simulink library "ddm"  (R2021b)
settings: Solver=VariableStepAuto  StartTime=0.0  StopTime=10.0  RelTol=1e-3
undefined symbols (not defined in the file or in its folder): ADDM_FrTMTqDev_X_Nm, ADDM_RrTMTqDev_X_Nm, ENUM_ADASACCSTA_ERROR, ENUM_ADASACCSTA_OFF, ENUM_ADASACCSTA_STANDBY, ENUM_ALLOWMOV_ALLOWREADY, ENUM_APS, ENUM_BRKSTA_ERROR, ENUM_BRKSTA_OFF, ENUM_BRKSTA_ON, ENUM_BRKSW_INVALID, ENUM_BRKSW_OFF, ENUM_BRKSW_ON, ENUM_CHGPREACTERRSTA_OBCPRE, ENUM_DCDCFAULTSTA_ANYFAULTLV1, ENUM_DCDCFAULTSTA_ANYFAULTLV2, ENUM_DRIVETRAIN_AWD, ENUM_DRIVETRAIN_FWD, ENUM_DRIVETRAIN_RWD, ENUM_EDUDRTSTA_NORMAL, ENUM_EPBSTA_APPLIED, ENUM_EPBSTA_RELEASED, ENUM_ESCAPSSta_APSUNAVAILABLE, ENUM_GEARACTUALPOSN_INVALID, ENUM_GEARACTUALPOSN_P, ENUM_HVBATTREADYPRE_READY, ENUM_MCUWARN_LV0, ENUM_MCUWARN_LV1, ENUM_MCUWARN_LV2, ENUM_MCUWARN_LV3, ENUM_MCUWARN_NOERROR, ENUM_OBCFAULTSTA_ANYFAULT, ENUM_PAS_R2F2, ENUM_PDFAULT_BATTPDFAIL, ENUM_PDFAULT_DCDCDISABLE, ENUM_PDFAULT_MCUDISABLE, ENUM_PDFAULT_MCUDISCHRG, ENUM_POWERSTA_OFF, ENUM_POWERSTA_ON, ENUM_POWERSTA_READY, ENUM_POWERSTA_STANDBY, ENUM_PRESSINDI_LOW, ENUM_PUFAULT_BATTUPFAIL, ENUM_PUFAULT_DCDCENABLEFAIL, ENUM_PUFAULT_PRECHRGCHKFAIL, ENUM_PUFAULT_SAFETYCHKFAIL, ENUM_PUSTATE_COMPLETED, ENUM_PWRSTASW_OFF, ENUM_PWRSTASW_OFFA, ENUM_PWRSTASW_OFFCHVCHRG, ENUM_PWRSTASW_OFFCLVCHRG, ENUM_PWRSTASW_ON, ENUM_PWRSTASW_ONHVCHRG, ENUM_PWRSTASW_READY, ENUM_PWRSTASW_STANDBY, ENUM_RAPSErrWarnSta_NORMAL, ENUM_RAPSErrWarnSta_RAPSERRLV1, ENUM_SHIFTCOMMAND_P, ENUM_SHIFTERERRSTA_PBUTTONFAILURE, ENUM_VEHMALFUNLV_2ND ... (+463)
libraries: hcu_lib x529, $bdroot x5, simulink x4
(part 13 of 25)

== system ddm/DDM/DDM/TQD/ESC1_DDM ==
  note: Diagnostics and Fault Handling
  note: Release Condition After Decision
  note: Release Condition After Decision
  note: Diagnostics and Fault Handling
  note: Diagnostics and Fault Handling
  note: Release Condition After Decision
  note: ESC1 CheckSum Error (ESC1CSErr)
  note: ESC1 Rolling Count Error (ESC1RCErr)
  note: ESC1 Lost Comm (ESC1NoCom)
  task_time_s : Inport
  VPMM_SysPwrSta_enum : Inport  Port=2
  No_CAN1_BUS_OFF : Inport  Port=3
  VDDM_ESC1NoCom_flg : Inport  Port=4
  VDDM_ESC1RCErr_flg : Inport  Port=5
  VDDM_ESC1CSErr_flg : Inport  Port=6
  DTC_clear_request : Inport  Port=7
  Constant{1,3..5,11,15,19..20,48} (9 alike) : Constant  Value=ENUM_PWRSTASW_OFF
  Constant10 : Constant  Value=KDDM_TQDDiagnosisOffSW_flg
  Constant101 : Constant  Value=KDDM_TQDDiagnosisOffSW_flg
  Constant102 : Constant  Value=ZERO_INT
  Constant12 : Constant  Value=FALSE
  Constant13 : Constant  Value=KDDM_ESC1RCErrDTC_cnt
  Constant14 : Constant  Value=KDDM_ESC1RCErrPassTO_s
  Constant16 : Constant  Value=KDDM_ESC1CSErrDTC_cnt
  Constant17 : Constant  Value=KDDM_TQDDiagnosisOffSW_flg
  Constant18 : Constant  Value=ENUM_PWRSTASW_STANDBY
  Constant2 : Constant  Value=KDDM_ESC1NoComDTC_cnt
  Constant25 : Constant  Value=KDDM_ESC1RCErrDetTO_s
  Constant27 : Constant  Value=FALSE
  Constant28 : Constant  Value=KDDM_ESC1NoComDTC_cnt
  Constant29 : Constant  Value=KDDM_ESC1NoComPassTO_s
  Constant30 : Constant  Value=KDDM_ESC1NoComDetTO_s
  Constant35 : Constant  Value=KDDM_ESC1RCErrPassTO_s
  Constant41 : Constant  Value=FALSE
  Constant42 : Constant  Value=KDDM_ESC1CSErrDTC_cnt
  Constant43 : Constant  Value=KDDM_ESC1CSErrPassTO_s
  Constant44 : Constant  Value=KDDM_ESC1CSErrDetTO_s
  Constant45 : Constant  Value=ZERO_INT
  Constant51 : Constant  Value=KDDM_ESC1CSErrPassTO_s
  Constant55 : Constant  Value=KDDM_ESC1NoComPassTO_s
  Constant6 : Constant  Value=KDDM_ESC1RCErrDTC_cnt
  Constant7 : Constant  Value=ZERO_INT
  Constant8 : Constant  Value=ENUM_PWRSTASW_STANDBY
  Constant9 : Constant  Value=ENUM_PWRSTASW_STANDBY
  DTC_Couter1 : hcu_lib/Basic_Blocks/DTC_Couter
  DTC_Couter2 : hcu_lib/Basic_Blocks/DTC_Couter
  DTC_Couter7 : hcu_lib/Basic_Blocks/DTC_Couter
  DTC_Info1 : hcu_lib/Basic_Blocks/DTC_Info
  DTC_Info2 : hcu_lib/Basic_Blocks/DTC_Info
  DTC_Info3 : hcu_lib/Basic_Blocks/DTC_Info
  Delay1 : Delay  DelayLength=1
  Delay2 : Delay  DelayLength=1
  Delay3 : Delay  DelayLength=1
  Equal{1,7,9..10,49..50} (6 alike) : RelationalOperator  Operator===  OutDataTypeStr=boolean  RndMeth=Simplest
  Equal{2..4,6,8,11} (6 alike) : RelationalOperator  Operator=~=  OutDataTypeStr=boolean  RndMeth=Simplest
  Equal15 : RelationalOperator  OutDataTypeStr=boolean  RndMeth=Simplest
  Equal20 : RelationalOperator  OutDataTypeStr=boolean  RndMeth=Simplest
  Equal21 : RelationalOperator  OutDataTypeStr=boolean  RndMeth=Simplest
  Logical Operator : Logic  Operator=OR  Inputs=3  AllPortsSameDT=off  OutDataTypeStr=boolean
  Logical Operator1 : Logic  Operator=OR  Inputs=4  AllPortsSameDT=off  OutDataTypeStr=boolean
  Logical Operator{11..13,19,26,30,37,41,45,53} (10 alike) : Logic  Operator=NOT  AllPortsSameDT=off  OutDataTypeStr=boolean
  Logical Operator{2,5,8..9,14,49} (6 alike) : Logic  AllPortsSameDT=off  OutDataTypeStr=boolean
  Logical Operator{28,32,43,46} (4 alike) : Logic  Inputs=4  AllPortsSameDT=off  OutDataTypeStr=boolean
  Logical Operator3 : Logic  Operator=OR  Inputs=4  AllPortsSameDT=off  OutDataTypeStr=boolean
  Logical Operator4 : Logic  Inputs=3  AllPortsSameDT=off  OutDataTypeStr=boolean
  Logical Operator50 : Logic  Inputs=3  AllPortsSameDT=off  OutDataTypeStr=boolean
  Logical Operator6 : Logic  Operator=OR  Inputs=4  AllPortsSameDT=off  OutDataTypeStr=boolean
  NOT1 : Logic  Operator=NOT  AllPortsSameDT=off  OutDataTypeStr=boolean
  NOT2 : Logic  Operator=NOT  AllPortsSameDT=off  OutDataTypeStr=boolean
  NOT3 : Logic  Operator=NOT  AllPortsSameDT=off  OutDataTypeStr=boolean
  Relational Operator1 : RelationalOperator  Operator=>  OutDataTypeStr=boolean  RndMeth=Simplest
  Relational Operator2 : RelationalOperator  Operator=>  OutDataTypeStr=boolean  RndMeth=Simplest
  Relational Operator3 : RelationalOperator  Operator=>  OutDataTypeStr=boolean  RndMeth=Simplest
  Switch1 : Switch  Criteria=u2 ~= 0
  Switch2 : Switch  Criteria=u2 ~= 0
  Switch3 : Switch  Criteria=u2 ~= 0
  Terminator : Terminator
  Terminator1 : Terminator
  Terminator2 : Terminator
  Test Detection Criteria2 : hcu_lib/Basic_Blocks/Test Detection Criteria
  Test Detection Criteria3 : hcu_lib/Basic_Blocks/Test Detection Criteria
  Test Detection Criteria4 : hcu_lib/Basic_Blocks/Test Detection Criteria
  Timer1 : hcu_lib/Basic_Blocks/Timer
  Timer3 : hcu_lib/Basic_Blocks/Timer
  Timer4 : hcu_lib/Basic_Blocks/Timer
  Unit Delay1 : UnitDelay  SampleTime=-1  HasFrameUpgradeWarning=on
  Unit Delay6 : UnitDelay  SampleTime=-1  HasFrameUpgradeWarning=on
  Unit Delay7 : UnitDelay  SampleTime=-1  HasFrameUpgradeWarning=on
  VDDM_ESC1NoComDTC_raw32 : Outport
  VDDM_ESC1RCErrDTC_raw32 : Outport  Port=2
  VDDM_ESC1CSErrDTC_raw32 : Outport  Port=3
  VDDM_ESC1NoComCFS_flg : Outport  Port=4
  VDDM_ESC1RCErrCFS_flg : Outport  Port=5
  VDDM_ESC1CSErrCFS_flg : Outport  Port=6
  VDDM_ESC1Err_flg : Outport  Port=7
  wires:
  [VPMM_SysPwrSta_enum] -> Equal8/1
  Constant15/1 -> Equal8/2
  Constant11/1 -> Equal11/2
  [VPMM_SysPwrSta_enum] -> Equal11/1
  Constant7/1 -> Relational Operator1/2
  Constant10/1 -> Logical Operator6/4
  [DTC_clear_request] -> Logical Operator6/2
  Unit Delay1/1 -> Equal10/1
  Logical Operator14/1 -> Logical Operator6/3
  Constant20/1 -> Equal10/2
  DTC_Couter2/2 -> Relational Operator1/1  "VDDM_ESC1CSErrDTC_cnt"
  Logical Operator2/1 -> Logical Operator6/1
  Equal10/1 -> Logical Operator2/1
  [VDDM_ESC1CSErrPass_flg] -> Logical Operator14/1
  Equal1/1 -> Logical Operator2/2
  Delay2/1 -> NOT2/1
  Constant16/1 -> DTC_Couter2/3
  NOT2/1 -> Logical Operator14/2
  Logical Operator6/1 -> [VDDM_ESC1CSErrCFSRls_flg]  "VDDM_ESC1CSErrCFSRls_flg"
  [VDDM_ESC1CSErrCFSRls_flg] -> DTC_Couter2/2
  [VDDM_ESC1CSErrDet_flg] -> DTC_Couter2/1
  Relational Operator1/1 -> Terminator2/1  "VDDM_ESC1CSErrDFS_flg"
  Constant8/1 -> Equal1/2
  DTC_Couter2/1 -> [VDDM_ESC1CSErrCFS_flg]  "VDDM_ESC1CSErrCFS_flg"
  [VPMM_SysPwrSta_enum] -> Equal1/1
  [VPMM_SysPwrSta_enum] -> Unit Delay1/1
  [VDDM_ESC1CSErrCFS_flg] -> Delay2/1
  [VPMM_SysPwrSta_enum] -> Equal4/1
  Constant5/1 -> Equal4/2
  [VPMM_SysPwrSta_enum] -> Equal3/1
  Constant4/1 -> Equal3/2
  NOT3/1 -> Logical Operator8/2
  [VDDM_ESC1RCErrPass_flg] -> Logical Operator8/1
  [VDDM_ESC1RCErrCFSRls_flg] -> DTC_Couter7/2
  Equal50/1 -> Logical Operator5/1
  [VDDM_ESC1RCErrCFS_flg] -> Delay3/1
  [VPMM_SysPwrSta_enum] -> Unit Delay7/1
  Equal49/1 -> Logical Operator5/2
  Delay3/1 -> NOT3/1
  Relational Operator3/1 -> Terminator1/1  "VDDM_ESC1RCErrDFS_flg"
  Constant9/1 -> Equal49/2
  DTC_Couter7/1 -> [VDDM_ESC1RCErrCFS_flg]  "VDDM_ESC1RCErrCFS_flg"
  [VDDM_ESC1RCErrDet_flg] -> DTC_Couter7/1
  Constant6/1 -> DTC_Couter7/3
  [VPMM_SysPwrSta_enum] -> Equal49/1
  Constant19/1 -> Equal50/2
  Unit Delay7/1 -> Equal50/1
  DTC_Couter7/2 -> Relational Operator3/1  "VDDM_ESC1RCErrDTC_cnt"
  Logical Operator8/1 -> Logical Operator3/3
  [DTC_clear_request] -> Logical Operator3/2
  Constant101/1 -> Logical Operator3/4
  Constant102/1 -> Relational Operator3/2
  Logical Operator3/1 -> [VDDM_ESC1RCErrCFSRls_flg]  "VDDM_ESC1RCErrCFSRls_flg"
  Logical Operator5/1 -> Logical Operator3/1
  [VPMM_SysPwrSta_enum] -> Unit Delay6/1
  [VDDM_ESC1NoComCFSRls_flg] -> DTC_Couter1/2
  Constant2/1 -> DTC_Couter1/3
  [DTC_clear_request] -> Logical Operator1/2
  [VDDM_ESC1NoComDet_flg] -> DTC_Couter1/1
  Constant45/1 -> Relational Operator2/2
  DTC_Couter1/2 -> Relational Operator2/1  "VDDM_ESC1NoComDTC_cnt"
  [VDDM_ESC1NoComPass_flg] -> Logical Operator49/1
  Logical Operator1/1 -> [VDDM_ESC1NoComCFSRls_flg]  "VDDM_ESC1NoComCFSRls_flg"
  Constant48/1 -> Equal9/2
  Equal9/1 -> Logical Operator9/1
  [VPMM_SysPwrSta_enum] -> Equal7/1
  Unit Delay6/1 -> Equal9/1
  DTC_Couter1/1 -> [VDDM_ESC1NoComCFS_flg]  "VDDM_ESC1NoComCFS_flg"
  Equal7/1 -> Logical Operator9/2
  [VDDM_ESC1NoComCFS_flg] -> Delay1/1
  Constant18/1 -> Equal7/2
  Logical Operator9/1 -> Logical Operator1/1
  NOT1/1 -> Logical Operator49/2
  Constant17/1 -> Logical Operator1/4
  Delay1/1 -> NOT1/1
  Logical Operator49/1 -> Logical Operator1/3
  Relational Operator2/1 -> Terminator/1  "VDDM_ESC1NoComDFS_flg"
  Constant1/1 -> Equal6/2
  [VPMM_SysPwrSta_enum] -> Equal6/1
  Constant3/1 -> Equal2/2
  [VPMM_SysPwrSta_enum] -> Equal2/1
  [VDDM_ESC1RCErrCFS_flg] -> VDDM_ESC1RCErrCFS_flg/1
  [VDDM_ESC1CSErrCFS_flg] -> VDDM_ESC1CSErrCFS_flg/1
  [VDDM_ESC1NoComCFS_flg] -> VDDM_ESC1NoComCFS_flg/1
  [VDDM_ESC1NoComCFS_flg] -> Logical Operator13/1
  Logical Operator13/1 -> Logical Operator43/4
  [VDDM_ESC1NoComCFS_flg] -> Logical Operator11/1
  Logical Operator11/1 -> Logical Operator28/4
  VDDM_ESC1CSErr_flg/1 -> [VDDM_ESC1CSErr_flg]
  VDDM_ESC1RCErr_flg/1 -> [VDDM_ESC1RCErr_flg]
  [VDDM_ESC1NoCom_flg] -> Logical Operator4/3
  Test Detection Criteria2/1 -> [VDDM_ESC1NoComDet_flg]  "VDDM_ESC1NoComDet_flg"
  Logical Operator37/1 -> Timer4/2
  Test Detection Criteria3/1 -> [VDDM_ESC1RCErrDet_flg]  "VDDM_ESC1RCErrDet_flg"
  [No_CAN1_BUS_OFF] -> Logical Operator32/2
  [No_CAN1_BUS_OFF] -> Logical Operator50/2
  [VDDM_ESC1NoCom_flg] -> Logical Operator53/1
  [VDDM_ESC1NoComPass_flg] -> DTC_Info1/2
  VDDM_ESC1NoCom_flg/1 -> [VDDM_ESC1NoCom_flg]
  Switch3/1 -> Test Detection Criteria2/1
  Timer4/1 -> Equal15/1
  Logical Operator41/1 -> Logical Operator32/4
  [VDDM_ESC1RCErr_flg] -> Logical Operator30/1
  Logical Operator19/1 -> Timer3/2
  Equal21/1 -> [VDDM_ESC1RCErrPass_flg]  "VDDM_ESC1RCErrPass_flg"
  Logical Operator43/1 -> Logical Operator37/1, Timer4/1
  Logical Operator53/1 -> Logical Operator50/3
  Logical Operator46/1 -> Switch1/3
  Constant44/1 -> Test Detection Criteria4/4
  [VDDM_ESC1CSErrCFS_flg] -> DTC_Info3/3
  Logical Operator26/1 -> Logical Operator46/4
  [VDDM_ESC1RCErrCFSRls_flg] -> Switch1/2
  [task_time_s] -> Timer4/3
  Constant12/1 -> Switch1/1
  Logical Operator12/1 -> Timer1/2
  [No_CAN1_BUS_OFF] -> Logical Operator4/2
  Logical Operator4/1 -> Switch3/3
  [task_time_s] -> Test Detection Criteria3/2
  [VDDM_ESC1RCErrDet_flg] -> DTC_Info2/1
  [task_time_s] -> Test Detection Criteria4/2
  Logical Operator28/1 -> Logical Operator12/1, Timer1/1
  Equal2/1 -> Logical Operator4/1
  DTC_Info1/1 -> VDDM_ESC1NoComDTC_raw32/1  "VDDM_ESC1NoComDTC_raw32"
  Constant13/1 -> Test Detection Criteria3/3
  Test Detection Criteria4/1 -> [VDDM_ESC1CSErrDet_flg]  "VDDM_ESC1CSErrDet_flg"
  Switch1/1 -> Test Detection Criteria3/1
  [VDDM_ESC1RCErr_flg] -> Logical Operator46/3
  Equal11/1 -> Logical Operator32/1
  [VDDM_ESC1CSErrDet_flg] -> DTC_Info3/1
  Logical Operator50/1 -> Timer3/1, Logical Operator19/1
  No_CAN1_BUS_OFF/1 -> [No_CAN1_BUS_OFF]
  [VDDM_ESC1NoComCFS_flg] -> Logical Operator26/1
  [DTC_clear_request] -> DTC_Info3/4
  Equal6/1 -> Logical Operator50/1
  [VDDM_ESC1CSErrCFSRls_flg] -> Switch2/2
  Constant42/1 -> Test Detection Criteria4/3
  [VDDM_ESC1NoComCFS_flg] -> Logical Operator41/1
  DTC_clear_request/1 -> [DTC_clear_request]
  [VDDM_ESC1RCErrCFS_flg] -> DTC_Info2/3
  Constant35/1 -> Timer1/4
  Logical Operator30/1 -> Logical Operator28/3
  Timer1/1 -> Equal21/1
  [VDDM_ESC1NoComDet_flg] -> DTC_Info1/1
  Equal4/1 -> Logical Operator28/1
  [No_CAN1_BUS_OFF] -> Logical Operator28/2
  Constant14/1 -> Equal21/2
  Logical Operator32/1 -> Switch2/3
  Equal20/1 -> [VDDM_ESC1NoComPass_flg]  "VDDM_ESC1NoComPass_flg"
  [VDDM_ESC1RCErrPass_flg] -> DTC_Info2/2
  [task_time_s] -> Timer1/3
  [VDDM_ESC1NoComCFSRls_flg] -> Switch3/2
  VPMM_SysPwrSta_enum/1 -> [VPMM_SysPwrSta_enum]
  Equal3/1 -> Logical Operator46/1
  Constant51/1 -> Timer4/4
  Switch2/1 -> Test Detection Criteria4/1
  [VDDM_ESC1CSErrPass_flg] -> DTC_Info3/2
  Equal15/1 -> [VDDM_ESC1CSErrPass_flg]  "VDDM_ESC1CSErrPass_flg"
  Constant43/1 -> Equal15/2
  Constant30/1 -> Test Detection Criteria2/4
  Constant28/1 -> Test Detection Criteria2/3
  [DTC_clear_request] -> DTC_Info2/4
  Constant25/1 -> Test Detection Criteria3/4
  [task_time_s] -> Timer3/3
  DTC_Info3/1 -> VDDM_ESC1CSErrDTC_raw32/1  "VDDM_ESC1CSErrDTC_raw32"
  [task_time_s] -> Test Detection Criteria2/2
  [VDDM_ESC1NoComCFS_flg] -> DTC_Info1/3
  [No_CAN1_BUS_OFF] -> Logical Operator43/2
  [VDDM_ESC1CSErr_flg] -> Logical Operator45/1
  DTC_Info2/1 -> VDDM_ESC1RCErrDTC_raw32/1  "VDDM_ESC1RCErrDTC_raw32"
  Equal8/1 -> Logical Operator43/1
  task_time_s/1 -> [task_time_s]
  Constant27/1 -> Switch3/1
  Constant29/1 -> Equal20/2
  Logical Operator45/1 -> Logical Operator43/3
  Constant41/1 -> Switch2/1
  [No_CAN1_BUS_OFF] -> Logical Operator46/2
  [DTC_clear_request] -> DTC_Info1/4
  Timer3/1 -> Equal20/1
  Constant55/1 -> Timer3/4
  [VDDM_ESC1CSErr_flg] -> Logical Operator32/3
  Logical Operator/1 -> VDDM_ESC1Err_flg/1  "VDDM_ESC1Err_flg"
  [VDDM_ESC1NoComCFS_flg] -> Logical Operator/1
  [VDDM_ESC1RCErrCFS_flg] -> Logical Operator/2
  [VDDM_ESC1CSErrCFS_flg] -> Logical Operator/3

== system ddm/DDM/DDM/TQD/ESC5_DDM ==
  note: Release Condition After Decision
  note: Diagnostics and Fault Handling
  note: Diagnostics and Fault Handling
  note: Release Condition After Decision
  note: Diagnostics and Fault Handling
  note: Release Condition After Decision
  note: ESC5 CheckSum Error (ESC5CSErr)
  note: ESC5 Rolling Count Error (ESC5RCErr)
  note: ESC5 Lost Comm (ESC5NoCom)
  task_time_s : Inport
  VPMM_SysPwrSta_enum : Inport  Port=2
  No_CAN1_BUS_OFF : Inport  Port=3
  VDDM_ESC5NoCom_flg : Inport  Port=4
  VDDM_ESC5RCErr_flg : Inport  Port=5
  VDDM_ESC5CSErr_flg : Inport  Port=6
  DTC_clear_request : Inport  Port=7
  Constant{1,3..5,11,15,18,22,48} (9 alike) : Constant  Value=ENUM_PWRSTASW_OFF
  Constant10 : Constant  Value=ENUM_PWRSTASW_STANDBY
  Constant101 : Constant  Value=KDDM_TQDDiagnosisOffSW_flg
  Constant102 : Constant  Value=ZERO_INT
  Constant12 : Constant  Value=FALSE
  Constant13 : Constant  Value=KDDM_ESC5RCErrDTC_cnt
  Constant14 : Constant  Value=KDDM_ESC5RCErrPassTO_s
  Constant17 : Constant  Value=KDDM_ESC5CSErrDTC_cnt
  Constant2 : Constant  Value=KDDM_ESC5NoComDTC_cnt
  Constant20 : Constant  Value=KDDM_TQDDiagnosisOffSW_flg
  Constant21 : Constant  Value=ENUM_PWRSTASW_STANDBY
  Constant25 : Constant  Value=KDDM_ESC5RCErrDetTO_s
  Constant27 : Constant  Value=FALSE
  Constant28 : Constant  Value=KDDM_ESC5NoComDTC_cnt
  Constant29 : Constant  Value=KDDM_ESC5NoComPassTO_s
  Constant30 : Constant  Value=KDDM_ESC5NoComDetTO_s
  Constant35 : Constant  Value=KDDM_ESC5RCErrPassTO_s
  Constant41 : Constant  Value=FALSE
  Constant42 : Constant  Value=KDDM_ESC5CSErrDTC_cnt
  Constant43 : Constant  Value=KDDM_ESC5CSErrPassTO_s
  Constant44 : Constant  Value=KDDM_ESC5CSErrDetTO_s
  Constant45 : Constant  Value=ZERO_INT
  Constant51 : Constant  Value=KDDM_ESC5CSErrPassTO_s
  Constant55 : Constant  Value=KDDM_ESC5NoComPassTO_s
  Constant6 : Constant  Value=KDDM_ESC5RCErrDTC_cnt
  Constant7 : Constant  Value=KDDM_TQDDiagnosisOffSW_flg
  Constant8 : Constant  Value=ZERO_INT
  Constant9 : Constant  Value=ENUM_PWRSTASW_STANDBY
  DTC_Couter1 : hcu_lib/Basic_Blocks/DTC_Couter
  DTC_Couter2 : hcu_lib/Basic_Blocks/DTC_Couter
  DTC_Couter7 : hcu_lib/Basic_Blocks/DTC_Couter
  DTC_Info1 : hcu_lib/Basic_Blocks/DTC_Info
  DTC_Info2 : hcu_lib/Basic_Blocks/DTC_Info
  DTC_Info3 : hcu_lib/Basic_Blocks/DTC_Info
  Delay1 : Delay  DelayLength=1
  Delay2 : Delay  DelayLength=1
  Delay3 : Delay  DelayLength=1
  Equal{1,7,19,23,49..50} (6 alike) : RelationalOperator  Operator===  OutDataTypeStr=boolean  RndMeth=Simplest
  Equal15 : RelationalOperator  OutDataTypeStr=boolean  RndMeth=Simplest
  Equal{2..6,8} (6 alike) : RelationalOperator  Operator=~=  OutDataTypeStr=boolean  RndMeth=Simplest
  Equal20 : RelationalOperator  OutDataTypeStr=boolean  RndMeth=Simplest
  Equal21 : RelationalOperator  OutDataTypeStr=boolean  RndMeth=Simplest
  Logical Operator : Logic  Operator=OR  Inputs=3  AllPortsSameDT=off  OutDataTypeStr=boolean
  Logical Operator1 : Logic  Operator=OR  Inputs=4  AllPortsSameDT=off  OutDataTypeStr=boolean
  Logical Operator{11..13,19,26,30,37,41,45,53} (10 alike) : Logic  Operator=NOT  AllPortsSameDT=off  OutDataTypeStr=boolean
  Logical Operator{2,5..6,8,54..55} (6 alike) : Logic  AllPortsSameDT=off  OutDataTypeStr=boolean
  Logical Operator{28,32,43,46} (4 alike) : Logic  Inputs=4  AllPortsSameDT=off  OutDataTypeStr=boolean
  Logical Operator3 : Logic  Operator=OR  Inputs=4  AllPortsSameDT=off  OutDataTypeStr=boolean
  Logical Operator4 : Logic  Inputs=3  AllPortsSameDT=off  OutDataTypeStr=boolean
  Logical Operator49 : Logic  Operator=OR  Inputs=4  AllPortsSameDT=off  OutDataTypeStr=boolean
  Logical Operator50 : Logic  Inputs=3  AllPortsSameDT=off  OutDataTypeStr=boolean
  NOT1 : Logic  Operator=NOT  AllPortsSameDT=off  OutDataTypeStr=boolean
  NOT2 : Logic  Operator=NOT  AllPortsSameDT=off  OutDataTypeStr=boolean
  NOT3 : Logic  Operator=NOT  AllPortsSameDT=off  OutDataTypeStr=boolean
  Relational Operator1 : RelationalOperator  Operator=>  OutDataTypeStr=boolean  RndMeth=Simplest
  Relational Operator2 : RelationalOperator  Operator=>  OutDataTypeStr=boolean  RndMeth=Simplest
  Relational Operator3 : RelationalOperator  Operator=>  OutDataTypeStr=boolean  RndMeth=Simplest
  Switch1 : Switch  Criteria=u2 ~= 0
  Switch2 : Switch  Criteria=u2 ~= 0
  Switch3 : Switch  Criteria=u2 ~= 0
  Terminator : Terminator
  Terminator1 : Terminator
  Terminator2 : Terminator
  Test Detection Criteria2 : hcu_lib/Basic_Blocks/Test Detection Criteria
  Test Detection Criteria3 : hcu_lib/Basic_Blocks/Test Detection Criteria
  Test Detection Criteria4 : hcu_lib/Basic_Blocks/Test Detection Criteria
  Timer1 : hcu_lib/Basic_Blocks/Timer
  Timer3 : hcu_lib/Basic_Blocks/Timer
  Timer4 : hcu_lib/Basic_Blocks/Timer
  Unit Delay1 : UnitDelay  SampleTime=-1  HasFrameUpgradeWarning=on
  Unit Delay6 : UnitDelay  SampleTime=-1  HasFrameUpgradeWarning=on
  Unit Delay7 : UnitDelay  SampleTime=-1  HasFrameUpgradeWarning=on
  VDDM_ESC5NoComDTC_raw32 : Outport
  VDDM_ESC5RCErrDTC_raw32 : Outport  Port=2
  VDDM_ESC5CSErrDTC_raw32 : Outport  Port=3
  VDDM_ESC5NoComCFS_flg : Outport  Port=4
  VDDM_ESC5RCErrCFS_flg : Outport  Port=5
  VDDM_ESC5CSErrCFS_flg : Outport  Port=6
  VDDM_ESC5Err_flg : Outport  Port=7
  wires:
  [VPMM_SysPwrSta_enum] -> Equal8/1
  Constant15/1 -> Equal8/2
  [VPMM_SysPwrSta_enum] -> Equal5/1
  Constant11/1 -> Equal5/2
  Equal7/1 -> Logical Operator2/1
  [VDDM_ESC5CSErrCFS_flg] -> Delay2/1
  Constant18/1 -> Equal7/2
  DTC_Couter2/2 -> Relational Operator1/1  "VDDM_ESC5CSErrDTC_cnt"
  [VDDM_ESC5CSErrCFSRls_flg] -> DTC_Couter2/2
  [DTC_clear_request] -> Logical Operator1/2
  Equal1/1 -> Logical Operator2/2
  Delay2/1 -> NOT2/1
  Logical Operator6/1 -> Logical Operator1/3
  Constant8/1 -> Relational Operator1/2
  Constant7/1 -> Logical Operator1/4
  Unit Delay1/1 -> Equal7/1
  Relational Operator1/1 -> Terminator2/1  "VDDM_ESC5CSErrDFS_flg"
  [VDDM_ESC5CSErrPass_flg] -> Logical Operator6/1
  DTC_Couter2/1 -> [VDDM_ESC5CSErrCFS_flg]  "VDDM_ESC5CSErrCFS_flg"
  [VPMM_SysPwrSta_enum] -> Unit Delay1/1
  Logical Operator2/1 -> Logical Operator1/1
  Constant10/1 -> Equal1/2
  NOT2/1 -> Logical Operator6/2
  [VPMM_SysPwrSta_enum] -> Equal1/1
  Constant17/1 -> DTC_Couter2/3
  Logical Operator1/1 -> [VDDM_ESC5CSErrCFSRls_flg]  "VDDM_ESC5CSErrCFSRls_flg"
  [VDDM_ESC5CSErrDet_flg] -> DTC_Couter2/1
  Equal49/1 -> Logical Operator5/2
  [VPMM_SysPwrSta_enum] -> Equal49/1
  NOT3/1 -> Logical Operator8/2
  DTC_Couter7/1 -> [VDDM_ESC5RCErrCFS_flg]  "VDDM_ESC5RCErrCFS_flg"
  Constant9/1 -> Equal49/2
  [VPMM_SysPwrSta_enum] -> Unit Delay7/1
  Equal50/1 -> Logical Operator5/1
  Relational Operator3/1 -> Terminator1/1  "VDDM_ESC5RCErrDFS_flg"
  [VDDM_ESC5RCErrPass_flg] -> Logical Operator8/1
  Logical Operator5/1 -> Logical Operator3/1
  [VDDM_ESC5RCErrCFS_flg] -> Delay3/1
  Logical Operator8/1 -> Logical Operator3/3
  Constant101/1 -> Logical Operator3/4
  [DTC_clear_request] -> Logical Operator3/2
  Constant102/1 -> Relational Operator3/2
  Constant6/1 -> DTC_Couter7/3
  [VDDM_ESC5RCErrDet_flg] -> DTC_Couter7/1
  Logical Operator3/1 -> [VDDM_ESC5RCErrCFSRls_flg]  "VDDM_ESC5RCErrCFSRls_flg"
  DTC_Couter7/2 -> Relational Operator3/1  "VDDM_ESC5RCErrDTC_cnt"
  Delay3/1 -> NOT3/1
  [VDDM_ESC5RCErrCFSRls_flg] -> DTC_Couter7/2
  Constant22/1 -> Equal50/2
  Unit Delay7/1 -> Equal50/1
  Constant5/1 -> Equal6/2
  [VPMM_SysPwrSta_enum] -> Equal6/1
  Constant4/1 -> Equal4/2
  [VPMM_SysPwrSta_enum] -> Equal4/1
  [VPMM_SysPwrSta_enum] -> Equal3/1
  Constant1/1 -> Equal3/2
  [VPMM_SysPwrSta_enum] -> Equal2/1
  Constant3/1 -> Equal2/2
  Equal19/1 -> Logical Operator55/2
  [VDDM_ESC5NoComPass_flg] -> Logical Operator54/1
  Constant2/1 -> DTC_Couter1/3
  [VDDM_ESC5NoComCFS_flg] -> Delay1/1
  DTC_Couter1/2 -> Relational Operator2/1  "VDDM_ESC5NoComDTC_cnt"
  DTC_Couter1/1 -> [VDDM_ESC5NoComCFS_flg]  "VDDM_ESC5NoComCFS_flg"
  Constant21/1 -> Equal19/2
  Equal23/1 -> Logical Operator55/1
  [VPMM_SysPwrSta_enum] -> Equal19/1
  [VDDM_ESC5NoComCFSRls_flg] -> DTC_Couter1/2
  [VDDM_ESC5NoComDet_flg] -> DTC_Couter1/1
  Constant48/1 -> Equal23/2
  Unit Delay6/1 -> Equal23/1
  Logical Operator49/1 -> [VDDM_ESC5NoComCFSRls_flg]  "VDDM_ESC5NoComCFSRls_flg"
  [DTC_clear_request] -> Logical Operator49/2
  Constant45/1 -> Relational Operator2/2
  Relational Operator2/1 -> Terminator/1  "VDDM_ESC5NoComDFS_flg"
  Logical Operator54/1 -> Logical Operator49/3
  Delay1/1 -> NOT1/1
  NOT1/1 -> Logical Operator54/2
  Constant20/1 -> Logical Operator49/4
  Logical Operator55/1 -> Logical Operator49/1
  [VPMM_SysPwrSta_enum] -> Unit Delay6/1
  [VDDM_ESC5CSErrCFS_flg] -> VDDM_ESC5CSErrCFS_flg/1
  [VDDM_ESC5RCErrCFS_flg] -> VDDM_ESC5RCErrCFS_flg/1
  [VDDM_ESC5NoComCFS_flg] -> VDDM_ESC5NoComCFS_flg/1
  [VDDM_ESC5NoComCFS_flg] -> Logical Operator13/1
  Logical Operator13/1 -> Logical Operator43/4
  [VDDM_ESC5NoComCFS_flg] -> Logical Operator11/1
  Logical Operator11/1 -> Logical Operator28/4
  VDDM_ESC5CSErr_flg/1 -> [VDDM_ESC5CSErr_flg]
  VDDM_ESC5RCErr_flg/1 -> [VDDM_ESC5RCErr_flg]
  [VDDM_ESC5NoCom_flg] -> Logical Operator4/3
  Test Detection Criteria2/1 -> [VDDM_ESC5NoComDet_flg]  "VDDM_ESC5NoComDet_flg"
  Logical Operator37/1 -> Timer4/2
  Test Detection Criteria3/1 -> [VDDM_ESC5RCErrDet_flg]  "VDDM_ESC5RCErrDet_flg"
  [No_CAN1_BUS_OFF] -> Logical Operator32/2
  [No_CAN1_BUS_OFF] -> Logical Operator50/2
  [VDDM_ESC5NoCom_flg] -> Logical Operator53/1
  [VDDM_ESC5NoComPass_flg] -> DTC_Info1/2
  VDDM_ESC5NoCom_flg/1 -> [VDDM_ESC5NoCom_flg]
  Switch3/1 -> Test Detection Criteria2/1
  Timer4/1 -> Equal15/1
  Logical Operator41/1 -> Logical Operator32/4
  [VDDM_ESC5RCErr_flg] -> Logical Operator30/1
  Logical Operator19/1 -> Timer3/2
  Equal21/1 -> [VDDM_ESC5RCErrPass_flg]  "VDDM_ESC5RCErrPass_flg"
  Logical Operator43/1 -> Logical Operator37/1, Timer4/1
  Logical Operator53/1 -> Logical Operator50/3
  Logical Operator46/1 -> Switch1/3
  Constant44/1 -> Test Detection Criteria4/4
  [VDDM_ESC5CSErrCFS_flg] -> DTC_Info3/3
  Logical Operator26/1 -> Logical Operator46/4
  [VDDM_ESC5RCErrCFSRls_flg] -> Switch1/2
  [task_time_s] -> Timer4/3
  Constant12/1 -> Switch1/1
  Logical Operator12/1 -> Timer1/2
  [No_CAN1_BUS_OFF] -> Logical Operator4/2
  Logical Operator4/1 -> Switch3/3
  [task_time_s] -> Test Detection Criteria3/2
  [VDDM_ESC5RCErrDet_flg] -> DTC_Info2/1
  [task_time_s] -> Test Detection Criteria4/2
  Logical Operator28/1 -> Logical Operator12/1, Timer1/1
  Equal2/1 -> Logical Operator4/1
  DTC_Info1/1 -> VDDM_ESC5NoComDTC_raw32/1  "VDDM_ESC5NoComDTC_raw32"
  Constant13/1 -> Test Detection Criteria3/3
  Test Detection Criteria4/1 -> [VDDM_ESC5CSErrDet_flg]  "VDDM_ESC5CSErrDet_flg"
  Switch1/1 -> Test Detection Criteria3/1
  [VDDM_ESC5RCErr_flg] -> Logical Operator46/3
  Equal5/1 -> Logical Operator32/1
  [VDDM_ESC5CSErrDet_flg] -> DTC_Info3/1
  Logical Operator50/1 -> Timer3/1, Logical Operator19/1
  No_CAN1_BUS_OFF/1 -> [No_CAN1_BUS_OFF]
  [VDDM_ESC5NoComCFS_flg] -> Logical Operator26/1
  [DTC_clear_request] -> DTC_Info3/4
  Equal3/1 -> Logical Operator50/1
  [VDDM_ESC5CSErrCFSRls_flg] -> Switch2/2
  Constant42/1 -> Test Detection Criteria4/3
  [VDDM_ESC5NoComCFS_flg] -> Logical Operator41/1
  DTC_clear_request/1 -> [DTC_clear_request]
  [VDDM_ESC5RCErrCFS_flg] -> DTC_Info2/3
  Constant35/1 -> Timer1/4
  Logical Operator30/1 -> Logical Operator28/3
  Timer1/1 -> Equal21/1
  [VDDM_ESC5NoComDet_flg] -> DTC_Info1/1
  Equal6/1 -> Logical Operator28/1
  [No_CAN1_BUS_OFF] -> Logical Operator28/2
  Constant14/1 -> Equal21/2
  Logical Operator32/1 -> Switch2/3
  Equal20/1 -> [VDDM_ESC5NoComPass_flg]  "VDDM_ESC5NoComPass_flg"
  [VDDM_ESC5RCErrPass_flg] -> DTC_Info2/2
  [task_time_s] -> Timer1/3
  [VDDM_ESC5NoComCFSRls_flg] -> Switch3/2
  VPMM_SysPwrSta_enum/1 -> [VPMM_SysPwrSta_enum]
  Equal4/1 -> Logical Operator46/1
  Constant51/1 -> Timer4/4
  Switch2/1 -> Test Detection Criteria4/1
  [VDDM_ESC5CSErrPass_flg] -> DTC_Info3/2
  Equal15/1 -> [VDDM_ESC5CSErrPass_flg]  "VDDM_ESC5CSErrPass_flg"
  Constant43/1 -> Equal15/2
  Constant30/1 -> Test Detection Criteria2/4
  Constant28/1 -> Test Detection Criteria2/3
  [DTC_clear_request] -> DTC_Info2/4
  Constant25/1 -> Test Detection Criteria3/4
  [task_time_s] -> Timer3/3
  DTC_Info3/1 -> VDDM_ESC5CSErrDTC_raw32/1  "VDDM_ESC5CSErrDTC_raw32"
  [task_time_s] -> Test Detection Criteria2/2
  [VDDM_ESC5NoComCFS_flg] -> DTC_Info1/3
  [No_CAN1_BUS_OFF] -> Logical Operator43/2
  [VDDM_ESC5CSErr_flg] -> Logical Operator45/1
  DTC_Info2/1 -> VDDM_ESC5RCErrDTC_raw32/1  "VDDM_ESC5RCErrDTC_raw32"
  Equal8/1 -> Logical Operator43/1
  task_time_s/1 -> [task_time_s]
  Constant27/1 -> Switch3/1
  Constant29/1 -> Equal20/2
  Logical Operator45/1 -> Logical Operator43/3
  Constant41/1 -> Switch2/1
  [No_CAN1_BUS_OFF] -> Logical Operator46/2
  [DTC_clear_request] -> DTC_Info1/4
  Timer3/1 -> Equal20/1
  Constant55/1 -> Timer3/4
  [VDDM_ESC5CSErr_flg] -> Logical Operator32/3
  [VDDM_ESC5RCErrCFS_flg] -> Logical Operator/2
  [VDDM_ESC5NoComCFS_flg] -> Logical Operator/1
  [VDDM_ESC5CSErrCFS_flg] -> Logical Operator/3
  Logical Operator/1 -> VDDM_ESC5Err_flg/1  "VDDM_ESC5Err_flg"
